simulink model "model_logistyczny"  (R2022b)
settings: Solver=VariableStepAuto  StartTime=0.0  StopTime=10.0  MaxStep=0.01  RelTol=1e-3
values from neighbouring files (symbols this model uses):
  alpha = alpha_warianty(i)    [logistyczny.m]
  K = K_base    (= 100)    [logistyczny.m]
  N0 = N0_base    (= 10)    [logistyczny.m]
  r = r_base    (= 0.5)    [logistyczny.m]
settings Model: Creator=matkw  LastModifiedBy=matkw

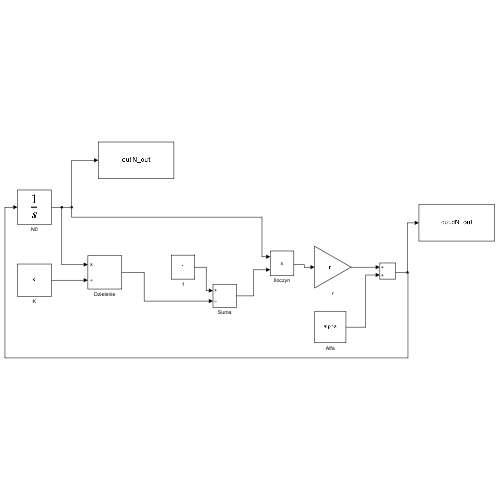
[thumbnail: Simulink's stored preview of the top-level diagram]
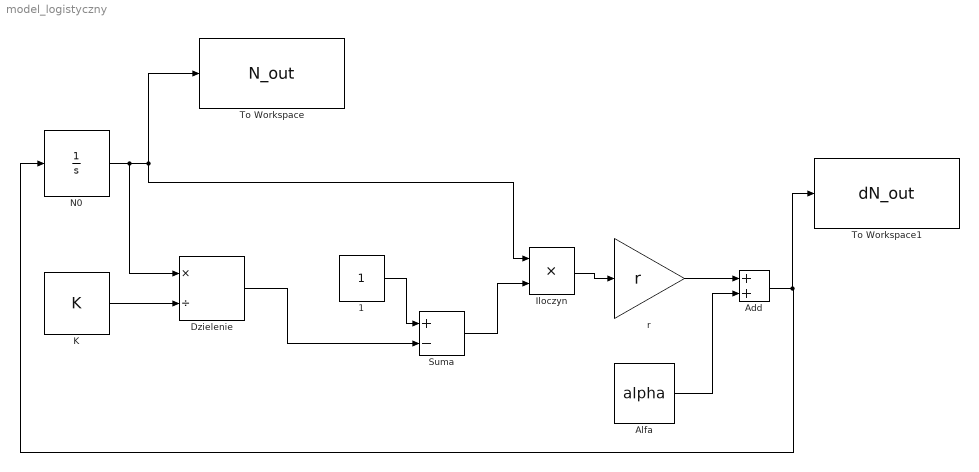
== system model_logistyczny ==
  1 : Constant
  Add : Sum
  Alfa : Constant  Value=alpha
  Dzielenie : Product  Inputs=*/
  Iloczyn : Product
  K : Constant  Value=K
  N0 : Integrator  InitialCondition=N0
  Suma : Sum  Inputs=+-
  To Workspace : ToWorkspace  VariableName=N_out  SampleTime=-1
  To Workspace1 : ToWorkspace  VariableName=dN_out  SampleTime=-1
  r : Gain  Gain=r
  wires:
  N0/1 -> Dzielenie/1, Iloczyn/1, To Workspace/1
  K/1 -> Dzielenie/2
  1/1 -> Suma/1
  Dzielenie/1 -> Suma/2
  Suma/1 -> Iloczyn/2
  Iloczyn/1 -> r/1
  r/1 -> Add/1
  Alfa/1 -> Add/2
  Add/1 -> To Workspace1/1, N0/1
